simulink model "sk_DepositosSS"  (Simulink 8.9)
settings: Solver=ode45  StartTime=0.0  StopTime=tsim  RelTol=1e-3  EnableMultiTasking=on
values from neighbouring files (symbols this model uses):
  h30 = 1    [Mod.m]
settings Model: Creator=ortega  LastModifiedBy=javi_  ExtModeTrigMode=oneshot  ExtModeArmWhenConnect=off
settings DataIOCC: LimitDataPoints=off
settings OptimizationCC: BlockReduction=off  BooleanDataType=off  ExpressionDepthLimit=2147483647  InitFltsAndDblsToZero=on
settings DebuggingCC: SaveWithParameterizedLinksMsg=none  SignalResolutionControl=TryResolveAllWithWarning  MultiTaskDSMMsg=warning  MultiTaskCondExecSysMsg=none
settings HardwareCC: TargetUnknown=on
settings GRTTargetCC: ModelReferenceCompliant=off  CompOptLevelCompliant=off  GeneratePreprocessorConditionals=Use local settings  MatFileLogging=off

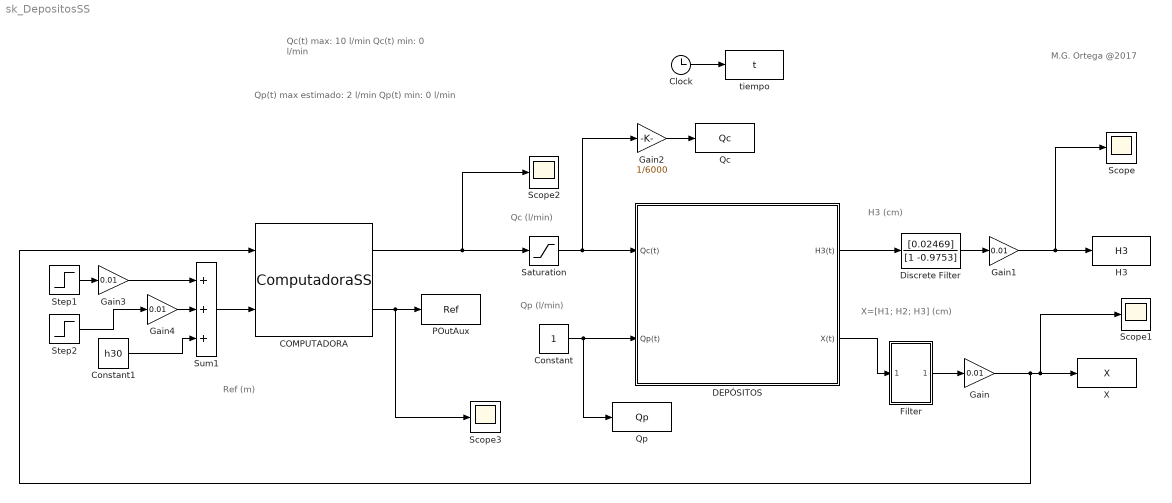
== system sk_DepositosSS ==
  note: Qc(t) max: 10 l/min
      | Qc(t) min:    0 l/min
  note: H3 (cm)
  note: Qc (l/min)
  note: Qp (l/min)
  note: Qp(t) max estimado: 2 l/min
      | Qp(t) min:    0 l/min
  note: M.G. Ortega @2017
  note: X=[H1; H2; H3] (cm)
  note: Ref (m)
  COMPUTADORA : S-Function  FunctionName=ComputadoraSS  Parameters=Tm  SFunctionDeploymentMode=off  EnableBusSupport=off  mask(Controlador){Tm=10}
      mask prompts: Tm "Tiempo de muestreo"
      mask help:
      | ENTRADAS:
      |   -  Estado del sistema: Xk = (Xk[0],Xk[1], Xk[2])
      |
      | SALIDAS:
      |   -  Señal de control: Ureal
      |   -  Puerto de salida auxiliar: POutAux
      mask Help:
      | Estos nombres no deberán ser modificados.
      | 
      |   El tiempo de muestreo se especifica mediante el único parámetro que se introduce desde Simulink
      |   En caso de ser utilizado en el código, su nombre será Tm.
      | 
      |   El alumno deberá modificar, en caso necesario, los siguiente ficheros:
      |   - Directivas.c
      |   - Declaraciones.c
      |   - Inicializaciones.c
      |   - Controlador.c
      | 
      | Autor: M.G. Ortega (2017)
      mask Display: image(imread('Computadora.jpg'))
  Clock : Clock
  Constant : Constant
  Constant1 : Constant  Value=h30
  DEPÓSITOS : Subsystem  mask{A1=40, A2=10, A3=30}
      mask prompts: A1 "Área del depósito 1 (cm^2)"; A2 "Área del depósito 2 (cm^2)"; A3 "Área del depósito 1 (cm^2)"
      mask help: SISTEMA CON TRES DEPÓSITOS EN SERIE
      mask Display: image(imread('Depositos.JPG'))
  Discrete Filter : DiscreteFilter  Numerator=[0.02469]  Denominator=[1 -0.9753]  SampleTime=0.01
  "Filter " : Subsystem
  Gain{,1,3..4} (4 alike) : Gain  Gain=0.01
  Gain2 : Gain  Gain=1/6000
  H3 : ToWorkspace  VariableName=H3
  POutAux : ToWorkspace  VariableName=Ref
  Qc : ToWorkspace  VariableName=Qc
  Qp : ToWorkspace  VariableName=Qp
  Saturation : Saturate  UpperLimit=10  LowerLimit=0
  Scope{,1..3} (4 alike) : Scope
  Step1 : Step  Time=150  After=20  SampleTime=0
  Step2 : Step  Time=250  After=-20  SampleTime=0
  Sum1 : Sum  Inputs=+++
  X : ToWorkspace  VariableName=X
  tiempo : ToWorkspace  VariableName=t  SampleTime=-1
  wires:
  Constant/1 -> DEPÓSITOS/2(Qp(t)), Qp/1
  Clock/1 -> tiempo/1
  COMPUTADORA/2 -> Scope3/1, POutAux/1
  Discrete Filter/1 -> Gain1/1
  DEPÓSITOS/1(H3(t)) -> Discrete Filter/1
  DEPÓSITOS/2(X(t)) -> "Filter "/1(In1)
  "Filter "/1(Out1) -> Gain/1
  COMPUTADORA/1 -> Saturation/1, Scope2/1
  Sum1/1 -> COMPUTADORA/2
  Step2/1 -> Gain4/1
  Step1/1 -> Gain3/1
  Gain/1 -> COMPUTADORA/1, X/1, Scope1/1
  Gain1/1 -> Scope/1, H3/1
  Constant1/1 -> Sum1/3
  Gain3/1 -> Sum1/1
  Gain4/1 -> Sum1/2
  Gain2/1 -> Qc/1
  Saturation/1 -> Gain2/1, DEPÓSITOS/1(Qc(t))

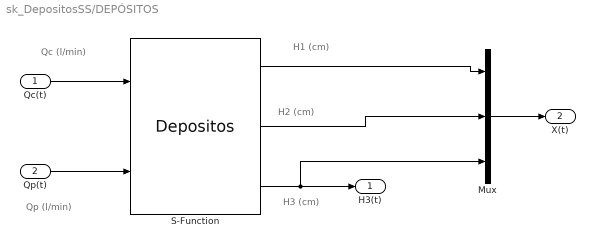
== system sk_DepositosSS/DEPÓSITOS ==
  note: H3 (cm)
  note: Qc (l/min)
  note: Qp (l/min)
  note: H2 (cm)
  note: H1 (cm)
  Qc(t) : Inport
  Qp(t) : Inport  Port=2
  Mux : Mux  Inputs=3
  S-Function : S-Function  FunctionName=Depositos  Parameters=A1;A2; A3  SFunctionDeploymentMode=off  EnableBusSupport=off
  H3(t) : Outport
  X(t) : Outport  Port=2
  wires:
  Qc(t)/1 -> S-Function/1
  Qp(t)/1 -> S-Function/2
  S-Function/3 -> H3(t)/1, Mux/3
  S-Function/1 -> Mux/1
  Mux/1 -> X(t)/1
  S-Function/2 -> Mux/2

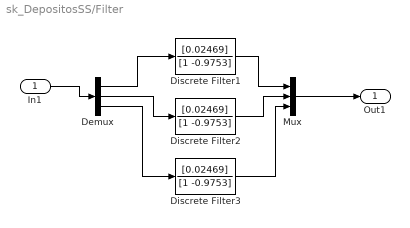
== system sk_DepositosSS/Filter  ==
  In1 : Inport
  Demux : Demux  Outputs=3
  Discrete Filter1 : DiscreteFilter  Numerator=[0.02469]  Denominator=[1 -0.9753]  SampleTime=0.01
  Discrete Filter2 : DiscreteFilter  Numerator=[0.02469]  Denominator=[1 -0.9753]  SampleTime=0.01
  Discrete Filter3 : DiscreteFilter  Numerator=[0.02469]  Denominator=[1 -0.9753]  SampleTime=0.01
  Mux : Mux  Inputs=3
  Out1 : Outport
  wires:
  Discrete Filter2/1 -> Mux/2
  Demux/3 -> Discrete Filter3/1
  Mux/1 -> Out1/1
  Discrete Filter1/1 -> Mux/1
  Discrete Filter3/1 -> Mux/3
  Demux/2 -> Discrete Filter2/1
  In1/1 -> Demux/1
  Demux/1 -> Discrete Filter1/1
